simulink model "numericaldifferentiation"  (Simulink 7.7)
settings: Solver=ode45  StartTime=0.0  StopTime=10.0  RelTol=1e-3
values from neighbouring files (symbols this model uses):
  A = [0 0 0.760636079841 108.52671545 0 0 -4.75493155594 137.180226521 1 0 -2.81921822895 14.6459088292 ... (16 elements, 4x4)]    [Equ_1_workspace.mat]    (also in StateFeedback_Controller_Observer_Design.m = [zeros(2,2),    eye(2,2); case1.mat; case2.mat = [0 0 0.760636079841 -110.04798761 0 0 -4.75493155594 -127.67)
  B = [0 0 0.100270957069 -0.520910116276]    [Equ_1_workspace.mat]    (also in StateFeedback_Controller_Observer_Design.m = [zeros(2,2); case1.mat; case2.mat = [0 0 0.100270957069 0.320368202138])
  K = [-5730.7096619 -3327.89921231 -1109.11662397 -307.639410763]    [Equ_1_workspace.mat]    (also in StateFeedback_Controller_Observer_Design.m = place(A,B,p); case1.mat; case2.mat = [3992.28365667 1479.45994307 676.936553485 -58.7389876522])
  Parameters = [11.8421 0.4216 0.1005 5.6072 1.1523 28.116 0.0111]    [Equ_1_workspace.mat]    (also in StateFeedback_Controller_Observer_Design.m = [11.8421; case1.mat; case2.mat)
  q1 = 1.57079632679    [Equ_1_workspace.mat]    (also in NonLinModel.m = x(1); StateFeedback_Controller_Observer_Design.m = 0.785398163397; case1.mat; case2.mat)
  q2 = 0    [Equ_1_workspace.mat]    (also in NonLinModel.m = x(2); StateFeedback_Controller_Observer_Design.m = 0.785398163397; case1.mat; case2.mat = 3.14159265359)
  T = 0.001    [Equ_1_workspace.mat]    (also in StateFeedback_Controller_Observer_Design.m; case1.mat; case2.mat)
  X0 = [1.67079632679 -0.2 0 0]    [Equ_1_workspace.mat]    (also in StateFeedback_Controller_Observer_Design.m = [q1+.1 q2-.2 0 0]; case1.mat; case2.mat = [1.67079632679 2.94159265359 0 0])
undefined symbols (not defined in the file or in its folder): DiscIntNeverNeededParam
settings Model: Creator=Sara  LastModifiedBy=Sara

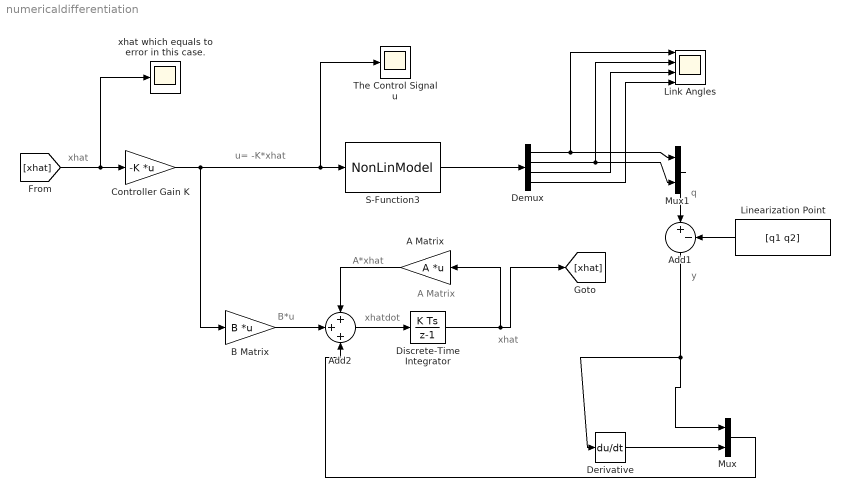
== system numericaldifferentiation ==
  note: q
  note: y
  note: B*u
  note: A Matrix
  note: A*xhat
  note: xhat
  note: u= -K*xhat
  note: xhatdot
  note: xhat
  A Matrix : Gain  Gain=A  Multiplication=Matrix(K*u)
  Add1 : Sum  Inputs=|+-
  Add2 : Sum  Inputs=+++
  B Matrix : Gain  Gain=B  Multiplication=Matrix(K*u)
  Controller Gain K : Gain  Gain=-K  Multiplication=Matrix(K*u)
  Demux : Demux
  Derivative : Derivative
  Discrete-Time Integrator : DiscreteIntegrator  InitialCondition=[0 0 0 0]'  SampleTime=T  ICPrevOutput=DiscIntNeverNeededParam  ICPrevScaledInput=DiscIntNeverNeededParam
  Linearization Point : Constant  Value=[q1 q2]
  Link Angles : Scope  NumInputPorts=4
      settings: YMin=-0.25~-5~-5~-5  YMax=1.75~5~5~5
  Mux : Mux  Inputs=2
  Mux1 : Mux  Inputs=2
  S-Function3 : S-Function  FunctionName=NonLinModel  Parameters=X0,Parameters  EnableBusSupport=off
  The Control Signal u : Scope
      settings: TimeRange=20  YMin=-110  YMax=110  SaveName=ScopeData2
  xhat which equals to error in this case. : Scope
      settings: YMin=-0.00024  YMax=-0.0001
  wires:
  Controller Gain K/1 -> B Matrix/1, The Control Signal u/1, S-Function3/1
  Mux1/1 -> Add1/1
  Demux/1 -> Mux1/1, Link Angles/1
  Demux/2 -> Mux1/2, Link Angles/2
  Add2/1 -> Discrete-Time Integrator/1
  Discrete-Time Integrator/1 -> A Matrix/1, [xhat]
  B Matrix/1 -> Add2/2
  A Matrix/1 -> Add2/1
  Linearization Point/1 -> Add1/2
  S-Function3/1 -> Demux/1
  [xhat] -> Controller Gain K/1, xhat which equals to error in this case./1
  Demux/3 -> Link Angles/3
  Demux/4 -> Link Angles/4
  Add1/1 -> Mux/1, Derivative/1
  Mux/1 -> Add2/3
  Derivative/1 -> Mux/2
